simulink model "Deployed_On_CPU2"  (R2020a)
settings: Solver=ode4  StartTime=0.0  StopTime=Inf  FixedStep=0.01  RelTol=1e-3  EnableMultiTasking=on
undefined symbols (not defined in the file): C28x, CPU1, CPU2
libraries: c280xlib x47, dspobslib x27, simulink x20, c2837xDlib x1
(part 1 of 3)
settings Model: ExtModeTrigDuration=8  Creator=NRPU  LastModifiedBy=NRPU
settings DataIOCC: SaveFormat=Array
settings OptimizationCC: DefaultUnderspecifiedDataType=single  EnhancedBackFolding=on  PassReuseOutputArgsAs=Individual arguments  MaxStackSize=1024  OptimizeBlockOrder=speed  DifferentSizesBufferReuse=on  OptimizationCustomize=off  DenormalBehavior=FlushToZero  EfficientTunableParamExpr=on
settings DebuggingCC: ParameterTunabilityLossMsg=error
settings HardwareCC: ProdBitPerChar=16  ProdBitPerInt=16  ProdBitPerPointer=32  ProdBitPerSizeT=32  ProdBitPerPtrDiffT=32  ProdLargestAtomicInteger=Integer  ProdLargestAtomicFloat=None  ProdWordSize=16  ProdLongLongMode=on  ProdHWDeviceType=Texas Instruments->C2000
settings SFSimCC: SimCustomHeaderCode="#include \"MadgwickAHRS.h\""  SimCustomInitializer=intialize();  SimUserSources=MadgwickAHRS.c  SimAnalyzeCustomCode=on  MATLABDynamicMemAlloc=off
settings RTWCC: SystemTargetFile=ert.tlc  HardwareBoard=TI Delfino F28379D LaunchPad  TLCOptions=-aInlineSetEventsForThisBaseRateFcn=TLC_FALSE -aSuppressMultiTaskScheduler=TLC_FALSE -aRateBasedStepFcn=1  TemplateMakefile=ert_default_tmf  RTWUseSimCustomCode=on  CustomHeaderCode="#include \"MadgwickAHRS.h\""  CustomSource=MadgwickAHRS.c  CustomInitializer=intialize();  Toolchain=Texas Instruments Code Composer Studio (C2000)  BuildConfiguration=Specify
settings CodeAppCC: ForceParamTrailComments=on  IgnoreCustomStorageClasses=off  OperatorAnnotations=on  SimulinkDataObjDesc=on  SFDataObjDesc=on  InsertBlockDesc=on
settings ERTTargetCC: CodeReplacementLibrary=TI C28x  SupportContinuousTime=on  ExtModeStaticAllocSize=10000

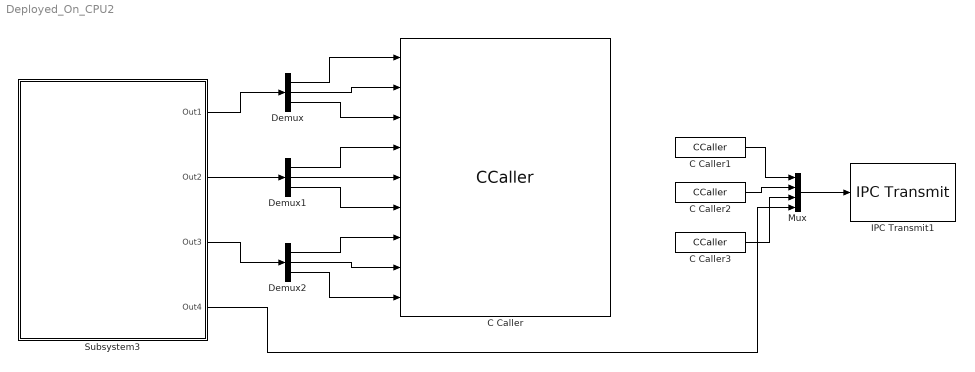
== system Deployed_On_CPU2 ==
  C Caller : CCaller  FunctionName=MadgwickQuaternionUpdate  PortSpecificationStruct="%)30     .    N!    8    (     @         %    \"     H    !     0         %  0 \"0    $    _    07)G3F%M90  4&]R=$YA;64 4V-O<&4     26YD97@     5'EP90      4VEZ90      27-';&]B86P   X    P    !@    @    $          4    (     0    ,    !         !   P!O=70 #@   #     &    \"     0         !0    @    !     P    $         $  # &]U=  .    .     8    (    !          %    \"     $    &     0         0   ...(+5398 chars)"
  C Caller1 : CCaller  FunctionName=roll  PortSpecificationStruct="%)30     .    & (   8    (     @         %    \"     $    !     0         %  0 \"0    $    _    07)G3F%M90  4&]R=$YA;64 4V-O<&4     26YD97@     5'EP90      4VEZ90      27-';&]B86P   X    P    !@    @    $          4    (     0    ,    !         !   P!O=70 #@   #     &    \"     0         !0    @    !     P    $         $  # &]U=  .    .     8    (    !          %    \"     $    &     0         0    !@   $]U='!U=   #@   #@    &    \"     8         !0    @    !     0    $         \"0    @               X    X    !@    @    $          4    (     0    8    !         !     &    <VEN9VQE   .    ,     8    (    !          %    \"     $    !     0         0  $ ,0    X    P    !@    @    ) @        4    (     0    $    !          (  0"
  C Caller2 : CCaller  FunctionName=pitch  PortSpecificationStruct="%)30     .    & (   8    (     @         %    \"     $    !     0         %  0 \"0    $    _    07)G3F%M90  4&]R=$YA;64 4V-O<&4     26YD97@     5'EP90      4VEZ90      27-';&]B86P   X    P    !@    @    $          4    (     0    ,    !         !   P!O=70 #@   #     &    \"     0         !0    @    !     P    $         $  # &]U=  .    .     8    (    !          %    \"     $    &     0         0    !@   $]U='!U=   #@   #@    &    \"     8         !0    @    !     0    $         \"0    @               X    X    !@    @    $          4    (     0    8    !         !     &    <VEN9VQE   .    ,     8    (    !          %    \"     $    !     0         0  $ ,0    X    P    !@    @    ) @        4    (     0    $    !          (  0"
  C Caller3 : CCaller  FunctionName=yaw  PortSpecificationStruct="%)30     .    & (   8    (     @         %    \"     $    !     0         %  0 \"0    $    _    07)G3F%M90  4&]R=$YA;64 4V-O<&4     26YD97@     5'EP90      4VEZ90      27-';&]B86P   X    P    !@    @    $          4    (     0    ,    !         !   P!O=70 #@   #     &    \"     0         !0    @    !     P    $         $  # &]U=  .    .     8    (    !          %    \"     $    &     0         0    !@   $]U='!U=   #@   #@    &    \"     8         !0    @    !     0    $         \"0    @               X    X    !@    @    $          4    (     0    8    !         !     &    <VEN9VQE   .    ,     8    (    !          %    \"     $    !     0         0  $ ,0    X    P    !@    @    ) @        4    (     0    $    !          (  0"
  Demux : Demux  Outputs=3
  Demux1 : Demux  Outputs=3
  Demux2 : Demux  Outputs=3
  IPC Transmit1 : c2837xDlib/IPC Transmit  blkParamProc=F2837x  SelectDestination=C28x (CPU1/CPU2)  SelectChannel=0  EnableBlocking=on
      settings: SourceProductBaseCode=TIC2000
  Mux : Mux
  Subsystem3 : Subsystem
      mask Display:
      | disp('GY-80')
      | port_label('Output',1,'Accelerometer','texmode','on')
      | port_label('Output',2,'Gyroscope','texmode','on')
      | port_label('Output',3,'Magnetometer','texmode','on')
      | port_label('Output',4,'MS5803','texmode','on')
  wires:
  Demux/1 -> C Caller/1
  Demux/2 -> C Caller/2
  Demux/3 -> C Caller/3
  Demux1/1 -> C Caller/4
  Demux1/2 -> C Caller/5
  Demux1/3 -> C Caller/6
  Demux2/1 -> C Caller/7
  Demux2/2 -> C Caller/8
  Demux2/3 -> C Caller/9
  C Caller1/1 -> Mux/1
  C Caller2/1 -> Mux/2
  C Caller3/1 -> Mux/3
  Subsystem3/1(Out1) -> Demux/1
  Subsystem3/2(Out2) -> Demux1/1
  Subsystem3/3(Out3) -> Demux2/1
  Subsystem3/4(Out4) -> Mux/4
  Mux/1 -> IPC Transmit1/1

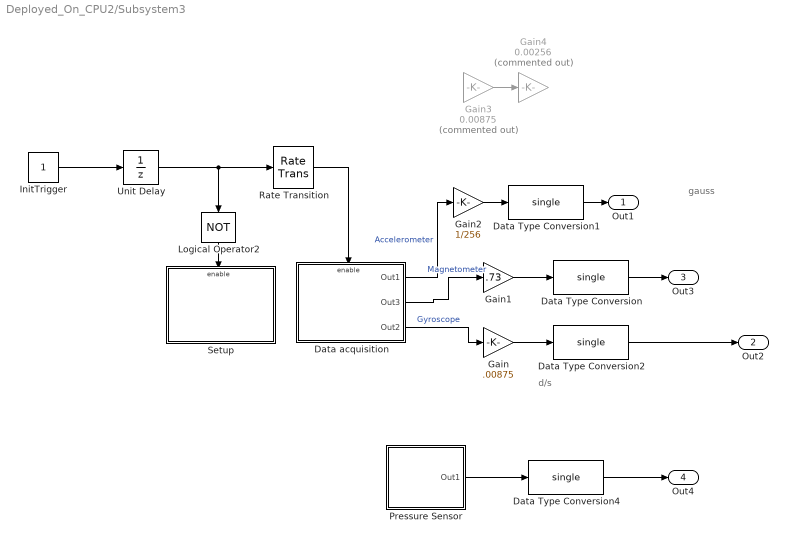
== system Deployed_On_CPU2/Subsystem3 ==
  note: gauss
  note: d/s
  Data Type Conversion{,1..2,4} (4 alike) : DataTypeConversion  OutDataTypeStr=single
  Data acquisition : Subsystem
  Gain : Gain  Gain=.00875  OutDataTypeStr=double
  Gain1 : Gain  Gain=.73  OutDataTypeStr=double
  Gain2 : Gain  Gain=1/256  OutDataTypeStr=double
  Gain3 : Gain  Commented=on  Gain=0.00875  OutDataTypeStr=int16
  Gain4 : Gain  Commented=on  Gain=0.00256  OutDataTypeStr=int16
  InitTrigger : Constant  Priority=10  OutDataTypeStr=uint16  SampleTime=0.01
  Logical Operator2 : Logic  Operator=NOT  AllPortsSameDT=off  OutDataTypeStr=boolean
  Pressure Sensor : Subsystem
  Rate Transition : RateTransition  OutPortSampleTime=0.01
  Setup : Subsystem  TreatAsAtomicUnit=on
  Unit Delay : UnitDelay  SampleTime=-1  HasFrameUpgradeWarning=on
  Out1 : Outport
  Out2 : Outport  Port=2
  Out3 : Outport  Port=3
  Out4 : Outport  Port=4
  wires:
  Rate Transition/1 -> Data acquisition/Enable
  Logical Operator2/1 -> Setup/Enable
  Unit Delay/1 -> Logical Operator2/1, Rate Transition/1
  InitTrigger/1 -> Unit Delay/1
  Data acquisition/1(Out1) -> Gain2/1  "Accelerometer"
  Data acquisition/3(Out2) -> Gain/1  "Gyroscope"
  Data acquisition/2(Out3) -> Gain1/1  "Magnetometer"
  Data Type Conversion/1 -> Out3/1
  Data Type Conversion1/1 -> Out1/1
  Gain1/1 -> Data Type Conversion/1
  Gain3/1 -> Gain4/1
  Gain2/1 -> Data Type Conversion1/1
  Gain/1 -> Data Type Conversion2/1
  Data Type Conversion2/1 -> Out2/1
  Pressure Sensor/1(Out1) -> Data Type Conversion4/1
  Data Type Conversion4/1 -> Out4/1

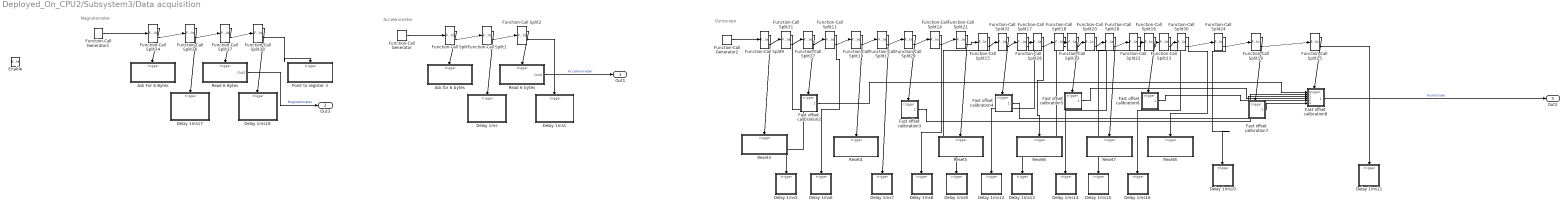
== system Deployed_On_CPU2/Subsystem3/Data acquisition ==
  note: Gyroscope
  note: Magnetometer
  note: Accelerometer
  Enable : EnablePort
  Ask For 6 Bytes : Subsystem  TreatAsAtomicUnit=on
  Ask for 6 bytes : Subsystem  TreatAsAtomicUnit=on
  Delay 1ms : Subsystem  TreatAsAtomicUnit=on
  Delay 1ms1 : Subsystem  TreatAsAtomicUnit=on
  Delay 1ms10 : Subsystem  TreatAsAtomicUnit=on
  Delay 1ms11 : Subsystem  TreatAsAtomicUnit=on
  Delay 1ms12 : Subsystem  TreatAsAtomicUnit=on
  Delay 1ms13 : Subsystem  TreatAsAtomicUnit=on
  Delay 1ms14 : Subsystem  TreatAsAtomicUnit=on
  Delay 1ms15 : Subsystem  TreatAsAtomicUnit=on
  Delay 1ms16 : Subsystem  TreatAsAtomicUnit=on
  Delay 1ms17 : Subsystem  TreatAsAtomicUnit=on
  Delay 1ms18 : Subsystem  TreatAsAtomicUnit=on
  Delay 1ms5 : Subsystem  TreatAsAtomicUnit=on
  Delay 1ms6 : Subsystem  TreatAsAtomicUnit=on
  Delay 1ms7 : Subsystem  TreatAsAtomicUnit=on
  Delay 1ms8 : Subsystem  TreatAsAtomicUnit=on
  Delay 1ms9 : Subsystem  TreatAsAtomicUnit=on
  Fast offset calibration2 : Subsystem  TreatAsAtomicUnit=on
  Fast offset calibration3 : Subsystem  TreatAsAtomicUnit=on
  Fast offset calibration4 : Subsystem  TreatAsAtomicUnit=on
  Fast offset calibration5 : Subsystem  TreatAsAtomicUnit=on
  Fast offset calibration6 : Subsystem  TreatAsAtomicUnit=on
  Fast offset calibration7 : Subsystem  TreatAsAtomicUnit=on
  Fast offset calibration8 : Subsystem  TreatAsAtomicUnit=on
  Function-Call Generator : simulink/Ports & Subsystems/Function-Call Generator  sample_time=0.01  numberOfIterations=1
  Function-Call Generator1 : simulink/Ports & Subsystems/Function-Call Generator  sample_time=0.01  numberOfIterations=1
  Function-Call Generator2 : simulink/Ports & Subsystems/Function-Call Generator  sample_time=0.01  numberOfIterations=1
  Function-Call Split{,1..2,9..32,34,36..38} (31 alike) : FunctionCallSplit  NumOutputPorts=2
  Ponit to register 3 : Subsystem  TreatAsAtomicUnit=on
  Read 6 Bytes : Subsystem  TreatAsAtomicUnit=on
  Read 6 bytes : Subsystem  TreatAsAtomicUnit=on
  Reset3 : Subsystem  TreatAsAtomicUnit=on
  Reset4 : Subsystem  TreatAsAtomicUnit=on
  Reset5 : Subsystem  TreatAsAtomicUnit=on
  Reset6 : Subsystem  TreatAsAtomicUnit=on
  Reset7 : Subsystem  TreatAsAtomicUnit=on
  Reset8 : Subsystem  TreatAsAtomicUnit=on
  Out1 : Outport
  Out3 : Outport  Port=2
  Out2 : Outport  Port=3
  wires:
  Function-Call Split19/2 -> Function-Call Split25/1
  Function-Call Split9/2 -> Function-Call Split31/1
  Function-Call Split27/1 -> Fast offset calibration2/Trigger
  Function-Call Split16/1 -> Fast offset calibration6/Trigger
  Function-Call Split10/2 -> Function-Call Split12/1
  Function-Call Split25/2 -> Delay 1ms11/Trigger
  Function-Call Split17/1 -> Delay 1ms12/Trigger
  Fast offset calibration7/1(Input) -> Fast offset calibration8/6(Input5)
  Fast offset calibration6/1(Input) -> Fast offset calibration8/5(Input4)
  Function-Call Split9/1 -> Reset3/Trigger
  Fast offset calibration2/1(Input) -> Fast offset calibration8/1(Input)
  Function-Call Split23/2 -> Function-Call Split30/1
  Fast offset calibration3/1(Input) -> Fast offset calibration8/2(Input1)
  Fast offset calibration4/1(Input) -> Fast offset calibration8/3(Input2)
  Function-Call Split32/2 -> Function-Call Split17/1
  Fast offset calibration8/1(Out2) -> Out2/1  "Gyroscope"
  Function-Call Split18/2 -> Function-Call Split13/1
  Function-Call Split24/1 -> Delay 1ms10/Trigger
  Function-Call Split10/1 -> Reset4/Trigger
  Function-Call Split29/2 -> Function-Call Split14/1
  Function-Call Split23/1 -> Delay 1ms16/Trigger
  Function-Call Split31/2 -> Function-Call Split27/1
  Function-Call Split17/2 -> Function-Call Split26/1
  Function-Call Split14/1 -> Delay 1ms8/Trigger
  Function-Call Split30/2 -> Function-Call Split24/1
  Function-Call Split21/1 -> Reset5/Trigger
  Function-Call Split30/1 -> Reset8/Trigger
  Function-Call Split11/2 -> Function-Call Split10/1
  Function-Call Split31/1 -> Delay 1ms5/Trigger
  Function-Call Split32/1 -> Fast offset calibration4/Trigger
  Fast offset calibration5/1(Input) -> Fast offset calibration8/4(Input3)
  Function-Call Split13/1 -> Fast offset calibration5/Trigger
  Function-Call Split15/2 -> Function-Call Split32/1
  Function-Call Split15/1 -> Delay 1ms9/Trigger
  Function-Call Split12/2 -> Function-Call Split29/1
  Function-Call Split20/2 -> Function-Call Split28/1
  Function-Call Split12/1 -> Delay 1ms7/Trigger
  Function-Call Split11/1 -> Delay 1ms6/Trigger
  Function-Call Split22/2 -> Function-Call Split16/1
  Function-Call Split26/1 -> Reset6/Trigger
  Function-Call Split28/2 -> Function-Call Split22/1
  Function-Call Split29/1 -> Fast offset calibration3/Trigger
  Function-Call Split20/1 -> Delay 1ms14/Trigger
  Function-Call Split22/1 -> Delay 1ms15/Trigger
  Function-Call Split13/2 -> Function-Call Split20/1
  Function-Call Split18/1 -> Delay 1ms13/Trigger
  Function-Call Split14/2 -> Function-Call Split21/1
  Function-Call Split21/2 -> Function-Call Split15/1
  Function-Call Split26/2 -> Function-Call Split18/1
  Function-Call Split19/1 -> Fast offset calibration7/Trigger
  Function-Call Split25/1 -> Fast offset calibration8/Trigger
  Function-Call Split27/2 -> Function-Call Split11/1
  Function-Call Split24/2 -> Function-Call Split19/1
  Function-Call Split28/1 -> Reset7/Trigger
  Function-Call Split16/2 -> Function-Call Split23/1
  Function-Call Split2/2 -> Delay 1ms1/Trigger
  Function-Call Split2/1 -> Read 6 bytes/Trigger
  Function-Call Split1/2 -> Function-Call Split2/1
  Function-Call Split/2 -> Function-Call Split1/1
  Function-Call Split1/1 -> Delay 1ms/Trigger
  Read 6 bytes/1(Out2) -> Out1/1  "Accelerometer"
  Function-Call Generator/1 -> Function-Call Split/1
  Function-Call Split/1 -> Ask for 6 bytes/Trigger
  Function-Call Split36/2 -> Function-Call Split37/1
  Function-Call Split37/2 -> Function-Call Split38/1
  Function-Call Split38/1 -> Delay 1ms18/Trigger
  Function-Call Generator1/1 -> Function-Call Split34/1
  Function-Call Split36/1 -> Delay 1ms17/Trigger
  Read 6 Bytes/1(Out2) -> Out3/1  "Magnetometer"
  Function-Call Split34/2 -> Function-Call Split36/1
  Function-Call Split37/1 -> Read 6 Bytes/Trigger
  Function-Call Split34/1 -> Ask For 6 Bytes/Trigger
  Function-Call Split38/2 -> Ponit to register 3/Trigger
  Function-Call Generator2/1 -> Function-Call Split9/1

== system Deployed_On_CPU2/Subsystem3/Pressure Sensor ==
  Data acquisition : Subsystem  Commented=on
  InitTrigger : Constant  Priority=10  Commented=on  OutDataTypeStr=uint16  SampleTime=0.01
  Logical Operator2 : Logic  Commented=on  Operator=NOT  AllPortsSameDT=off  OutDataTypeStr=boolean
  Rate Transition : RateTransition  Commented=on  OutPortSampleTime=0.01
  Setup : Subsystem  Commented=on  TreatAsAtomicUnit=on
  Unit Delay : UnitDelay  Commented=on  SampleTime=-1  HasFrameUpgradeWarning=on
  Out1 : Outport
  wires:
  Unit Delay/1 -> Logical Operator2/1, Rate Transition/1
  Data acquisition/1(Out1) -> Out1/1
  Rate Transition/1 -> Data acquisition/Enable
  InitTrigger/1 -> Unit Delay/1
  Logical Operator2/1 -> Setup/Enable

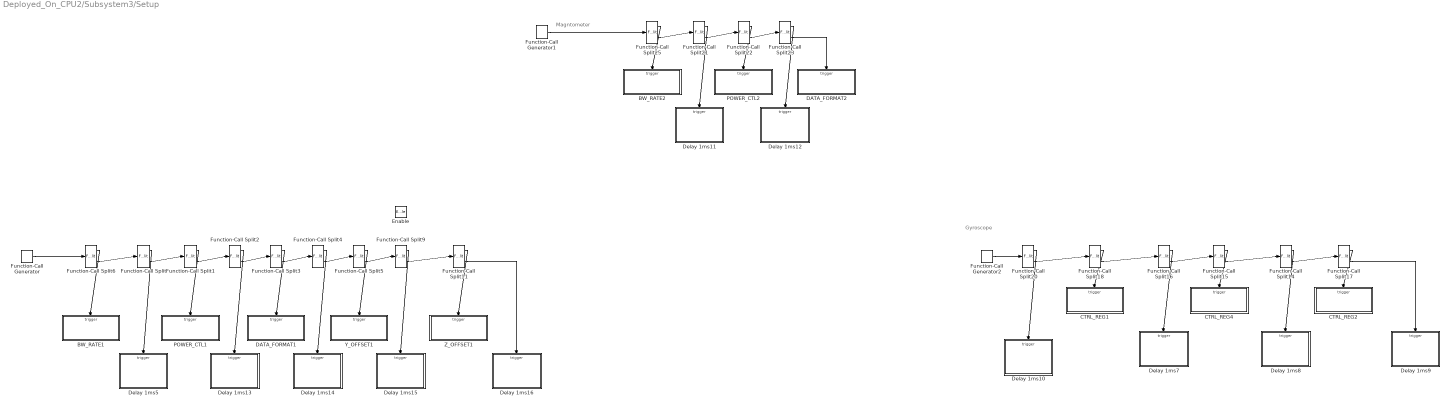
== system Deployed_On_CPU2/Subsystem3/Setup ==
  note: Gyroscope
  note: Magntometer
  Enable : EnablePort
  BW_RATE1 : Subsystem  TreatAsAtomicUnit=on
  BW_RATE2 : Subsystem  TreatAsAtomicUnit=on
  CTRL_REG1 : Subsystem  TreatAsAtomicUnit=on
  CTRL_REG2 : Subsystem  TreatAsAtomicUnit=on
  CTRL_REG4 : Subsystem  TreatAsAtomicUnit=on
  DATA_FORMAT1 : Subsystem  TreatAsAtomicUnit=on
  DATA_FORMAT2 : Subsystem  TreatAsAtomicUnit=on
  Delay 1ms10 : Subsystem  TreatAsAtomicUnit=on
  Delay 1ms11 : Subsystem  TreatAsAtomicUnit=on
  Delay 1ms12 : Subsystem  TreatAsAtomicUnit=on
  Delay 1ms13 : Subsystem  TreatAsAtomicUnit=on
  Delay 1ms14 : Subsystem  TreatAsAtomicUnit=on
  Delay 1ms15 : Subsystem  TreatAsAtomicUnit=on
  Delay 1ms16 : Subsystem  TreatAsAtomicUnit=on
  Delay 1ms5 : Subsystem  TreatAsAtomicUnit=on
  Delay 1ms7 : Subsystem  TreatAsAtomicUnit=on
  Delay 1ms8 : Subsystem  TreatAsAtomicUnit=on
  Delay 1ms9 : Subsystem  TreatAsAtomicUnit=on
  Function-Call Generator : simulink/Ports & Subsystems/Function-Call Generator  sample_time=0.01  numberOfIterations=1
  Function-Call Generator1 : simulink/Ports & Subsystems/Function-Call Generator  sample_time=0.01  numberOfIterations=1
  Function-Call Generator2 : simulink/Ports & Subsystems/Function-Call Generator  sample_time=0.01  numberOfIterations=1
  Function-Call Split{,1..6,9,11,14..18,20..23,25} (19 alike) : FunctionCallSplit  NumOutputPorts=2
  POWER_CTL1 : Subsystem  TreatAsAtomicUnit=on
  POWER_CTL2 : Subsystem  TreatAsAtomicUnit=on
  Y_OFFSET1 : Subsystem  TreatAsAtomicUnit=on
  Z_OFFSET1 : Subsystem  TreatAsAtomicUnit=on
  wires:
  Function-Call Split20/1 -> Delay 1ms10/Trigger
  Function-Call Split17/2 -> Delay 1ms9/Trigger
  Function-Call Split15/1 -> CTRL_REG4/Trigger
  Function-Call Split15/2 -> Function-Call Split14/1
  Function-Call Split16/2 -> Function-Call Split15/1
  Function-Call Split17/1 -> CTRL_REG2/Trigger
  Function-Call Split14/2 -> Function-Call Split17/1
  Function-Call Split18/1 -> CTRL_REG1/Trigger
  Function-Call Split20/2 -> Function-Call Split18/1
  Function-Call Split14/1 -> Delay 1ms8/Trigger
  Function-Call Split16/1 -> Delay 1ms7/Trigger
  Function-Call Split18/2 -> Function-Call Split16/1
  Function-Call Split3/2 -> Function-Call Split4/1
  Function-Call Split4/2 -> Function-Call Split5/1
  Function-Call Split2/2 -> Function-Call Split3/1
  Function-Call Split/2 -> Function-Call Split1/1
  Function-Call Split1/2 -> Function-Call Split2/1
  Function-Call Split23/2 -> DATA_FORMAT2/Trigger
  Function-Call Split21/2 -> Function-Call Split22/1
  Function-Call Split21/1 -> Delay 1ms11/Trigger
  Function-Call Split23/1 -> Delay 1ms12/Trigger
  Function-Call Split22/2 -> Function-Call Split23/1
  Function-Call Split25/2 -> Function-Call Split21/1
  Function-Call Split25/1 -> BW_RATE2/Trigger
  Function-Call Split22/1 -> POWER_CTL2/Trigger
  Function-Call Generator1/1 -> Function-Call Split25/1
  Function-Call Generator2/1 -> Function-Call Split20/1
  Function-Call Split5/2 -> Function-Call Split9/1
  Function-Call Split9/2 -> Function-Call Split11/1
  Function-Call Split/1 -> Delay 1ms5/Trigger
  Function-Call Split4/1 -> Delay 1ms14/Trigger
  Function-Call Split9/1 -> Delay 1ms15/Trigger
  Function-Call Split2/1 -> Delay 1ms13/Trigger
  Function-Call Split11/2 -> Delay 1ms16/Trigger
  Function-Call Split1/1 -> POWER_CTL1/Trigger
  Function-Call Split3/1 -> DATA_FORMAT1/Trigger
  Function-Call Split5/1 -> Y_OFFSET1/Trigger
  Function-Call Split11/1 -> Z_OFFSET1/Trigger
  Function-Call Split6/1 -> BW_RATE1/Trigger
  Function-Call Split6/2 -> Function-Call Split/1
  Function-Call Generator/1 -> Function-Call Split6/1

== system Deployed_On_CPU2/Subsystem3/Data acquisition/Ask For 6 Bytes ==
  function : TriggerPort  TriggerType=function-call  VariantControl=Variant
  Data Read Adress : Constant  Priority=10  Value=hex2dec('06')  OutDataTypeStr=uint8  SampleTime=-1
  I2C Transmit : c280xlib/I2C Transmit  Priority=20  selectModule=I2C_A  addrFormat=7-Bit addressing  saSource=Specify via dialog  SAR=hex2dec('1E')  bitCount=8  STP=on  RM=off  STR=on
      settings: SourceProductBaseCode=TIC2000
  Terminator : Terminator
  wires:
  Data Read Adress/1 -> I2C Transmit/1
  I2C Transmit/1 -> Terminator/1

== system Deployed_On_CPU2/Subsystem3/Data acquisition/Ask for 6 bytes ==
  function : TriggerPort  TriggerType=function-call  VariantControl=Variant
  Data Read Adress : Constant  Priority=10  Value=hex2dec('32')  OutDataTypeStr=uint8  SampleTime=-1
  I2C Transmit : c280xlib/I2C Transmit  Priority=20  selectModule=I2C_A  addrFormat=7-Bit addressing  saSource=Specify via dialog  SAR=83  bitCount=8  STP=on  RM=off  STR=on
      settings: SourceProductBaseCode=TIC2000
  Terminator : Terminator
  wires:
  I2C Transmit/1 -> Terminator/1
  Data Read Adress/1 -> I2C Transmit/1

== system Deployed_On_CPU2/Subsystem3/Data acquisition/Delay 1ms ==
  function : TriggerPort  TriggerType=function-call  VariantControl=Variant
  System Outputs : Subsystem  mask(System Outputs){ShowInLibBrowser=0}
      mask prompts: ShowInLibBrowser "Simulink:masks:CustCodeMaskParam1_MP"
      settings: CopyFcn=cccopyfcn(gcb)  OpenFcn=ccopenfcn('System Outputs Function')
      mask Help: eval('feval(''rtwprivate'',''rtwhelpview'',''rtw_sys_outputs_block'')');
      mask Display: disp('System\nOutputs');

== system Deployed_On_CPU2/Subsystem3/Data acquisition/Delay 1ms1 ==
  function : TriggerPort  TriggerType=function-call  VariantControl=Variant
  System Outputs : Subsystem  mask(System Outputs){ShowInLibBrowser=0}
      mask prompts: ShowInLibBrowser "Simulink:masks:CustCodeMaskParam1_MP"
      settings: CopyFcn=cccopyfcn(gcb)  OpenFcn=ccopenfcn('System Outputs Function')
      mask Help: eval('feval(''rtwprivate'',''rtwhelpview'',''rtw_sys_outputs_block'')');
      mask Display: disp('System\nOutputs');

== system Deployed_On_CPU2/Subsystem3/Data acquisition/Delay 1ms10 ==
  function : TriggerPort  TriggerType=function-call  VariantControl=Variant
  System Outputs : Subsystem  mask(System Outputs){ShowInLibBrowser=0}
      mask prompts: ShowInLibBrowser "Simulink:masks:CustCodeMaskParam1_MP"
      settings: CopyFcn=cccopyfcn(gcb)  OpenFcn=ccopenfcn('System Outputs Function')
      mask Help: eval('feval(''rtwprivate'',''rtwhelpview'',''rtw_sys_outputs_block'')');
      mask Display: disp('System\nOutputs');

== system Deployed_On_CPU2/Subsystem3/Data acquisition/Delay 1ms11 ==
  function : TriggerPort  TriggerType=function-call  VariantControl=Variant
  System Outputs : Subsystem  mask(System Outputs){ShowInLibBrowser=0}
      mask prompts: ShowInLibBrowser "Simulink:masks:CustCodeMaskParam1_MP"
      settings: CopyFcn=cccopyfcn(gcb)  OpenFcn=ccopenfcn('System Outputs Function')
      mask Help: eval('feval(''rtwprivate'',''rtwhelpview'',''rtw_sys_outputs_block'')');
      mask Display: disp('System\nOutputs');

== system Deployed_On_CPU2/Subsystem3/Data acquisition/Delay 1ms12 ==
  function : TriggerPort  TriggerType=function-call  VariantControl=Variant
  System Outputs : Subsystem  mask(System Outputs){ShowInLibBrowser=0}
      mask prompts: ShowInLibBrowser "Simulink:masks:CustCodeMaskParam1_MP"
      settings: CopyFcn=cccopyfcn(gcb)  OpenFcn=ccopenfcn('System Outputs Function')
      mask Help: eval('feval(''rtwprivate'',''rtwhelpview'',''rtw_sys_outputs_block'')');
      mask Display: disp('System\nOutputs');

== system Deployed_On_CPU2/Subsystem3/Data acquisition/Delay 1ms13 ==
  function : TriggerPort  TriggerType=function-call  VariantControl=Variant
  System Outputs : Subsystem  mask(System Outputs){ShowInLibBrowser=0}
      mask prompts: ShowInLibBrowser "Simulink:masks:CustCodeMaskParam1_MP"
      settings: CopyFcn=cccopyfcn(gcb)  OpenFcn=ccopenfcn('System Outputs Function')
      mask Help: eval('feval(''rtwprivate'',''rtwhelpview'',''rtw_sys_outputs_block'')');
      mask Display: disp('System\nOutputs');

== system Deployed_On_CPU2/Subsystem3/Data acquisition/Delay 1ms14 ==
  function : TriggerPort  TriggerType=function-call  VariantControl=Variant
  System Outputs : Subsystem  mask(System Outputs){ShowInLibBrowser=0}
      mask prompts: ShowInLibBrowser "Simulink:masks:CustCodeMaskParam1_MP"
      settings: CopyFcn=cccopyfcn(gcb)  OpenFcn=ccopenfcn('System Outputs Function')
      mask Help: eval('feval(''rtwprivate'',''rtwhelpview'',''rtw_sys_outputs_block'')');
      mask Display: disp('System\nOutputs');

== system Deployed_On_CPU2/Subsystem3/Data acquisition/Delay 1ms15 ==
  function : TriggerPort  TriggerType=function-call  VariantControl=Variant
  System Outputs : Subsystem  mask(System Outputs){ShowInLibBrowser=0}
      mask prompts: ShowInLibBrowser "Simulink:masks:CustCodeMaskParam1_MP"
      settings: CopyFcn=cccopyfcn(gcb)  OpenFcn=ccopenfcn('System Outputs Function')
      mask Help: eval('feval(''rtwprivate'',''rtwhelpview'',''rtw_sys_outputs_block'')');
      mask Display: disp('System\nOutputs');

== system Deployed_On_CPU2/Subsystem3/Data acquisition/Delay 1ms16 ==
  function : TriggerPort  TriggerType=function-call  VariantControl=Variant
  System Outputs : Subsystem  mask(System Outputs){ShowInLibBrowser=0}
      mask prompts: ShowInLibBrowser "Simulink:masks:CustCodeMaskParam1_MP"
      settings: CopyFcn=cccopyfcn(gcb)  OpenFcn=ccopenfcn('System Outputs Function')
      mask Help: eval('feval(''rtwprivate'',''rtwhelpview'',''rtw_sys_outputs_block'')');
      mask Display: disp('System\nOutputs');

== system Deployed_On_CPU2/Subsystem3/Data acquisition/Delay 1ms17 ==
  function : TriggerPort  TriggerType=function-call  VariantControl=Variant
  System Outputs : Subsystem  mask(System Outputs){ShowInLibBrowser=0}
      mask prompts: ShowInLibBrowser "Simulink:masks:CustCodeMaskParam1_MP"
      settings: CopyFcn=cccopyfcn(gcb)  OpenFcn=ccopenfcn('System Outputs Function')
      mask Help: eval('feval(''rtwprivate'',''rtwhelpview'',''rtw_sys_outputs_block'')');
      mask Display: disp('System\nOutputs');

== system Deployed_On_CPU2/Subsystem3/Data acquisition/Delay 1ms18 ==
  function : TriggerPort  TriggerType=function-call  VariantControl=Variant
  System Outputs : Subsystem  mask(System Outputs){ShowInLibBrowser=0}
      mask prompts: ShowInLibBrowser "Simulink:masks:CustCodeMaskParam1_MP"
      settings: CopyFcn=cccopyfcn(gcb)  OpenFcn=ccopenfcn('System Outputs Function')
      mask Help: eval('feval(''rtwprivate'',''rtwhelpview'',''rtw_sys_outputs_block'')');
      mask Display: disp('System\nOutputs');

== system Deployed_On_CPU2/Subsystem3/Data acquisition/Delay 1ms5 ==
  function : TriggerPort  TriggerType=function-call  VariantControl=Variant
  System Outputs : Subsystem  mask(System Outputs){ShowInLibBrowser=0}
      mask prompts: ShowInLibBrowser "Simulink:masks:CustCodeMaskParam1_MP"
      settings: CopyFcn=cccopyfcn(gcb)  OpenFcn=ccopenfcn('System Outputs Function')
      mask Help: eval('feval(''rtwprivate'',''rtwhelpview'',''rtw_sys_outputs_block'')');
      mask Display: disp('System\nOutputs');

== system Deployed_On_CPU2/Subsystem3/Data acquisition/Delay 1ms6 ==
  function : TriggerPort  TriggerType=function-call  VariantControl=Variant
  System Outputs : Subsystem  mask(System Outputs){ShowInLibBrowser=0}
      mask prompts: ShowInLibBrowser "Simulink:masks:CustCodeMaskParam1_MP"
      settings: CopyFcn=cccopyfcn(gcb)  OpenFcn=ccopenfcn('System Outputs Function')
      mask Help: eval('feval(''rtwprivate'',''rtwhelpview'',''rtw_sys_outputs_block'')');
      mask Display: disp('System\nOutputs');

== system Deployed_On_CPU2/Subsystem3/Data acquisition/Delay 1ms7 ==
  function : TriggerPort  TriggerType=function-call  VariantControl=Variant
  System Outputs : Subsystem  mask(System Outputs){ShowInLibBrowser=0}
      mask prompts: ShowInLibBrowser "Simulink:masks:CustCodeMaskParam1_MP"
      settings: CopyFcn=cccopyfcn(gcb)  OpenFcn=ccopenfcn('System Outputs Function')
      mask Help: eval('feval(''rtwprivate'',''rtwhelpview'',''rtw_sys_outputs_block'')');
      mask Display: disp('System\nOutputs');

== system Deployed_On_CPU2/Subsystem3/Data acquisition/Delay 1ms8 ==
  function : TriggerPort  TriggerType=function-call  VariantControl=Variant
  System Outputs : Subsystem  mask(System Outputs){ShowInLibBrowser=0}
      mask prompts: ShowInLibBrowser "Simulink:masks:CustCodeMaskParam1_MP"
      settings: CopyFcn=cccopyfcn(gcb)  OpenFcn=ccopenfcn('System Outputs Function')
      mask Help: eval('feval(''rtwprivate'',''rtwhelpview'',''rtw_sys_outputs_block'')');
      mask Display: disp('System\nOutputs');

== system Deployed_On_CPU2/Subsystem3/Data acquisition/Delay 1ms9 ==
  function : TriggerPort  TriggerType=function-call  VariantControl=Variant
  System Outputs : Subsystem  mask(System Outputs){ShowInLibBrowser=0}
      mask prompts: ShowInLibBrowser "Simulink:masks:CustCodeMaskParam1_MP"
      settings: CopyFcn=cccopyfcn(gcb)  OpenFcn=ccopenfcn('System Outputs Function')
      mask Help: eval('feval(''rtwprivate'',''rtwhelpview'',''rtw_sys_outputs_block'')');
      mask Display: disp('System\nOutputs');

== system Deployed_On_CPU2/Subsystem3/Data acquisition/Fast offset calibration2 ==
  function : TriggerPort  TriggerType=function-call  VariantControl=Variant
  I2C Receive1 : c280xlib/I2C Receive  Priority=10  selectModule=I2C_A  addrFormat=7-Bit addressing  saSource=Specify via dialog  SAR=hex2dec('69')  bitCount=8  dataLength=1  initValue=0  NACK=off  STP=on  STR=on  sampleTime=-1  dataType=uint8
      settings: SourceProductBaseCode=TIC2000
  Terminator : Terminator
  Input : Outport
  wires:
  I2C Receive1/1 -> Input/1
  I2C Receive1/2 -> Terminator/1

== system Deployed_On_CPU2/Subsystem3/Data acquisition/Fast offset calibration3 ==
  function : TriggerPort  TriggerType=function-call  VariantControl=Variant
  I2C Receive1 : c280xlib/I2C Receive  Priority=10  selectModule=I2C_A  addrFormat=7-Bit addressing  saSource=Specify via dialog  SAR=hex2dec('69')  bitCount=8  dataLength=1  initValue=0  NACK=off  STP=on  STR=on  sampleTime=-1  dataType=uint8
      settings: SourceProductBaseCode=TIC2000
  Terminator : Terminator
  Input : Outport
  wires:
  I2C Receive1/2 -> Terminator/1
  I2C Receive1/1 -> Input/1

== system Deployed_On_CPU2/Subsystem3/Data acquisition/Fast offset calibration4 ==
  function : TriggerPort  TriggerType=function-call  VariantControl=Variant
  I2C Receive1 : c280xlib/I2C Receive  Priority=10  selectModule=I2C_A  addrFormat=7-Bit addressing  saSource=Specify via dialog  SAR=hex2dec('69')  bitCount=8  dataLength=1  initValue=0  NACK=off  STP=on  STR=on  sampleTime=-1  dataType=uint8
      settings: SourceProductBaseCode=TIC2000
  Terminator : Terminator
  Input : Outport
  wires:
  I2C Receive1/2 -> Terminator/1
  I2C Receive1/1 -> Input/1

== system Deployed_On_CPU2/Subsystem3/Data acquisition/Fast offset calibration5 ==
  function : TriggerPort  TriggerType=function-call  VariantControl=Variant
  I2C Receive1 : c280xlib/I2C Receive  Priority=10  selectModule=I2C_A  addrFormat=7-Bit addressing  saSource=Specify via dialog  SAR=hex2dec('69')  bitCount=8  dataLength=1  initValue=0  NACK=off  STP=on  STR=on  sampleTime=-1  dataType=uint8
      settings: SourceProductBaseCode=TIC2000
  Terminator : Terminator
  Input : Outport
  wires:
  I2C Receive1/2 -> Terminator/1
  I2C Receive1/1 -> Input/1

== system Deployed_On_CPU2/Subsystem3/Data acquisition/Fast offset calibration6 ==
  function : TriggerPort  TriggerType=function-call  VariantControl=Variant
  I2C Receive1 : c280xlib/I2C Receive  Priority=10  selectModule=I2C_A  addrFormat=7-Bit addressing  saSource=Specify via dialog  SAR=hex2dec('69')  bitCount=8  dataLength=1  initValue=0  NACK=off  STP=on  STR=on  sampleTime=-1  dataType=uint8
      settings: SourceProductBaseCode=TIC2000
  Terminator : Terminator
  Input : Outport
  wires:
  I2C Receive1/2 -> Terminator/1
  I2C Receive1/1 -> Input/1

== system Deployed_On_CPU2/Subsystem3/Data acquisition/Fast offset calibration7 ==
  function : TriggerPort  TriggerType=function-call  VariantControl=Variant
  I2C Receive1 : c280xlib/I2C Receive  Priority=10  selectModule=I2C_A  addrFormat=7-Bit addressing  saSource=Specify via dialog  SAR=hex2dec('69')  bitCount=8  dataLength=1  initValue=0  NACK=off  STP=on  STR=on  sampleTime=-1  dataType=uint8
      settings: SourceProductBaseCode=TIC2000
  Terminator : Terminator
  Input : Outport
  wires:
  I2C Receive1/2 -> Terminator/1
  I2C Receive1/1 -> Input/1

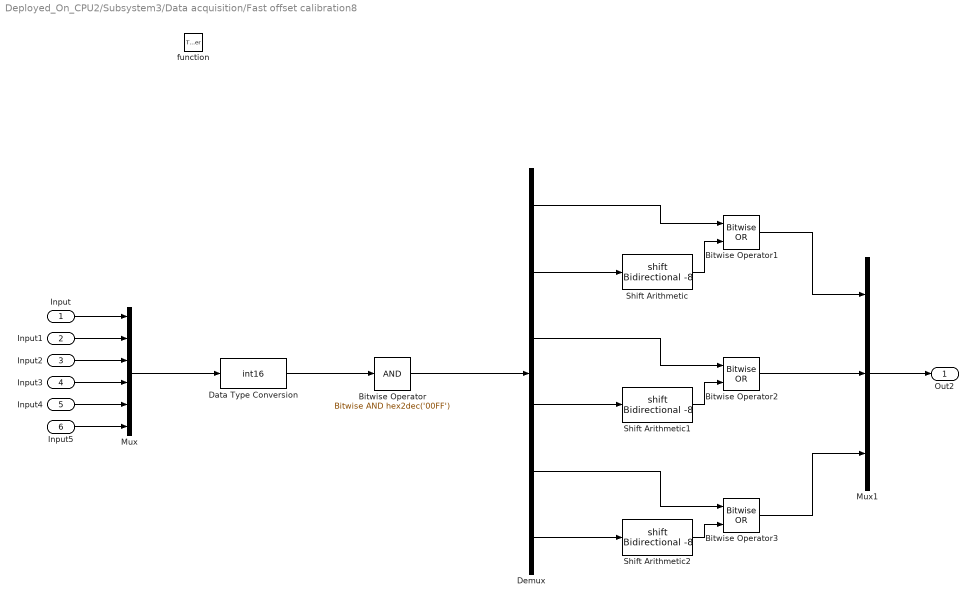
== system Deployed_On_CPU2/Subsystem3/Data acquisition/Fast offset calibration8 ==
  Input : Inport
  Input1 : Inport  Port=2
  Input2 : Inport  Port=3
  Input3 : Inport  Port=4
  Input4 : Inport  Port=5
  Input5 : Inport  Port=6
  function : TriggerPort  TriggerType=function-call  VariantControl=Variant
  Bitwise Operator : simulink/Logic and Bit Operations/Bitwise Operator  logicop=AND  UseBitMask=on  BitMask=hex2dec('00FF')  BitMaskRealWorld=Stored Integer
  Bitwise Operator1 : simulink/Logic and Bit Operations/Bitwise Operator  logicop=OR  UseBitMask=off  NumInputPorts=2  BitMask=bin2dec('11011001')  BitMaskRealWorld=Stored Integer
  Bitwise Operator2 : simulink/Logic and Bit Operations/Bitwise Operator  logicop=OR  UseBitMask=off  NumInputPorts=2  BitMask=bin2dec('11011001')  BitMaskRealWorld=Stored Integer
  Bitwise Operator3 : simulink/Logic and Bit Operations/Bitwise Operator  logicop=OR  UseBitMask=off  NumInputPorts=2  BitMask=bin2dec('11011001')  BitMaskRealWorld=Stored Integer
  Data Type Conversion : DataTypeConversion  OutDataTypeStr=int16  ConvertRealWorld=Stored Integer (SI)
  Demux : Demux  Outputs=6
  Mux : Mux  Inputs=6
  Mux1 : Mux  Inputs=3
  Shift Arithmetic : ArithShift  BitShiftNumber=-8
  Shift Arithmetic1 : ArithShift  BitShiftNumber=-8
  Shift Arithmetic2 : ArithShift  BitShiftNumber=-8
  Out2 : Outport
  wires:
  Demux/6 -> Shift Arithmetic2/1
  Input5/1 -> Mux/6
  Input4/1 -> Mux/5
  Input3/1 -> Mux/4
  Input2/1 -> Mux/3
  Input1/1 -> Mux/2
  Input/1 -> Mux/1
  Shift Arithmetic1/1 -> Bitwise Operator2/2
  Bitwise Operator2/1 -> Mux1/2
  Bitwise Operator3/1 -> Mux1/3
  Bitwise Operator1/1 -> Mux1/1
  Mux1/1 -> Out2/1
  Shift Arithmetic/1 -> Bitwise Operator1/2
  Demux/3 -> Bitwise Operator2/1
  Bitwise Operator/1 -> Demux/1
  Shift Arithmetic2/1 -> Bitwise Operator3/2
  Demux/5 -> Bitwise Operator3/1
  Demux/1 -> Bitwise Operator1/1
  Demux/2 -> Shift Arithmetic/1
  Data Type Conversion/1 -> Bitwise Operator/1
  Demux/4 -> Shift Arithmetic1/1
  Mux/1 -> Data Type Conversion/1

== system Deployed_On_CPU2/Subsystem3/Data acquisition/Ponit to register 3 ==
  function : TriggerPort  TriggerType=function-call  VariantControl=Variant
  Data Read Adress : Constant  Priority=10  Value=hex2dec('03')  OutDataTypeStr=uint8  SampleTime=-1
  I2C Transmit : c280xlib/I2C Transmit  Priority=20  selectModule=I2C_A  addrFormat=7-Bit addressing  saSource=Specify via dialog  SAR=hex2dec('1E')  bitCount=8  STP=on  RM=off  STR=on
      settings: SourceProductBaseCode=TIC2000
  Terminator : Terminator
  wires:
  I2C Transmit/1 -> Terminator/1
  Data Read Adress/1 -> I2C Transmit/1

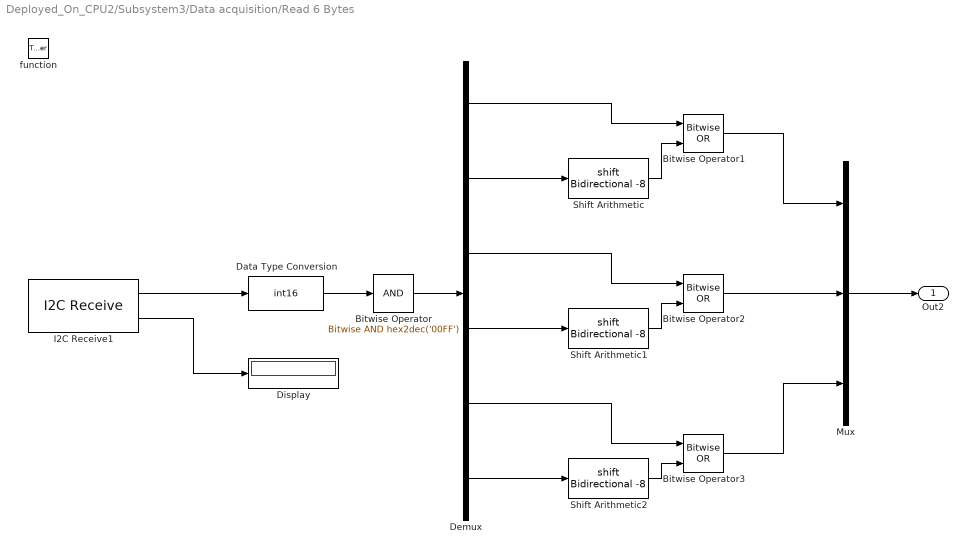
== system Deployed_On_CPU2/Subsystem3/Data acquisition/Read 6 Bytes ==
  function : TriggerPort  TriggerType=function-call  VariantControl=Variant
  Bitwise Operator : simulink/Logic and Bit Operations/Bitwise Operator  logicop=AND  UseBitMask=on  BitMask=hex2dec('00FF')  BitMaskRealWorld=Stored Integer
  Bitwise Operator1 : simulink/Logic and Bit Operations/Bitwise Operator  logicop=OR  UseBitMask=off  NumInputPorts=2  BitMask=bin2dec('11011001')  BitMaskRealWorld=Stored Integer
  Bitwise Operator2 : simulink/Logic and Bit Operations/Bitwise Operator  logicop=OR  UseBitMask=off  NumInputPorts=2  BitMask=bin2dec('11011001')  BitMaskRealWorld=Stored Integer
  Bitwise Operator3 : simulink/Logic and Bit Operations/Bitwise Operator  logicop=OR  UseBitMask=off  NumInputPorts=2  BitMask=bin2dec('11011001')  BitMaskRealWorld=Stored Integer
  Data Type Conversion : DataTypeConversion  OutDataTypeStr=int16  ConvertRealWorld=Stored Integer (SI)
  Demux : Demux  Outputs=6
  Display : Display
  I2C Receive1 : c280xlib/I2C Receive  Priority=10  selectModule=I2C_A  addrFormat=7-Bit addressing  saSource=Specify via dialog  SAR=hex2dec('1E')  bitCount=8  dataLength=6  initValue=0  NACK=off  STP=on  STR=on  sampleTime=-1  dataType=uint8
      settings: SourceProductBaseCode=TIC2000
  Mux : Mux  Inputs=3
  Shift Arithmetic : ArithShift  BitShiftNumber=-8
  Shift Arithmetic1 : ArithShift  BitShiftNumber=-8
  Shift Arithmetic2 : ArithShift  BitShiftNumber=-8
  Out2 : Outport
  wires:
  I2C Receive1/1 -> Data Type Conversion/1
  I2C Receive1/2 -> Display/1
  Data Type Conversion/1 -> Bitwise Operator/1
  Bitwise Operator/1 -> Demux/1
  Demux/5 -> Bitwise Operator3/1
  Demux/1 -> Bitwise Operator1/1
  Demux/6 -> Shift Arithmetic2/1
  Demux/4 -> Shift Arithmetic1/1
  Demux/2 -> Shift Arithmetic/1
  Shift Arithmetic2/1 -> Bitwise Operator3/2
  Shift Arithmetic1/1 -> Bitwise Operator2/2
  Demux/3 -> Bitwise Operator2/1
  Mux/1 -> Out2/1
  Shift Arithmetic/1 -> Bitwise Operator1/2
  Bitwise Operator2/1 -> Mux/2
  Bitwise Operator3/1 -> Mux/3
  Bitwise Operator1/1 -> Mux/1

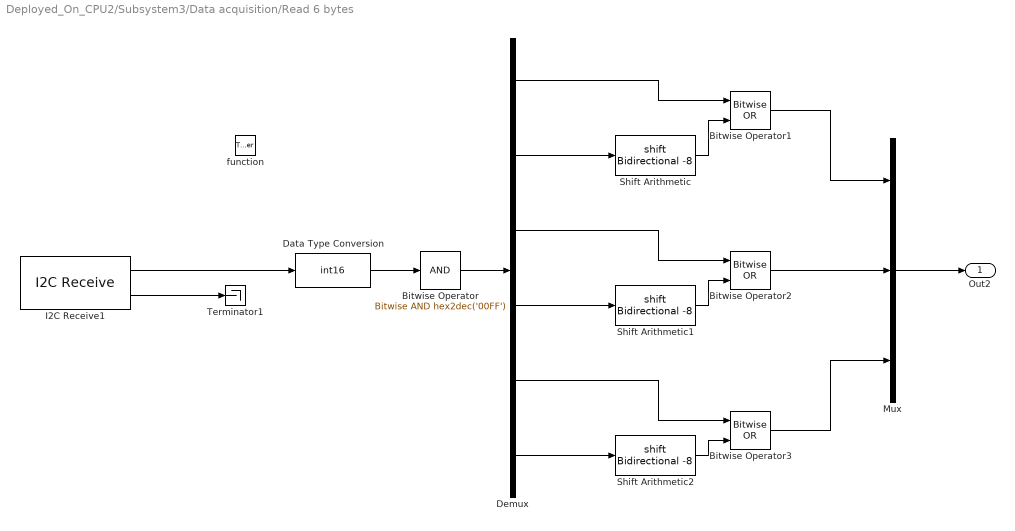
== system Deployed_On_CPU2/Subsystem3/Data acquisition/Read 6 bytes ==
  function : TriggerPort  TriggerType=function-call  VariantControl=Variant
  Bitwise Operator : simulink/Logic and Bit Operations/Bitwise Operator  logicop=AND  UseBitMask=on  BitMask=hex2dec('00FF')  BitMaskRealWorld=Stored Integer
  Bitwise Operator1 : simulink/Logic and Bit Operations/Bitwise Operator  logicop=OR  UseBitMask=off  NumInputPorts=2  BitMask=bin2dec('11011001')  BitMaskRealWorld=Stored Integer
  Bitwise Operator2 : simulink/Logic and Bit Operations/Bitwise Operator  logicop=OR  UseBitMask=off  NumInputPorts=2  BitMask=bin2dec('11011001')  BitMaskRealWorld=Stored Integer
  Bitwise Operator3 : simulink/Logic and Bit Operations/Bitwise Operator  logicop=OR  UseBitMask=off  NumInputPorts=2  BitMask=bin2dec('11011001')  BitMaskRealWorld=Stored Integer
  Data Type Conversion : DataTypeConversion  OutDataTypeStr=int16  ConvertRealWorld=Stored Integer (SI)
  Demux : Demux  Outputs=6
  I2C Receive1 : c280xlib/I2C Receive  Priority=10  selectModule=I2C_A  addrFormat=7-Bit addressing  saSource=Specify via dialog  SAR=83  bitCount=8  dataLength=6  initValue=0  NACK=off  STP=on  STR=on  sampleTime=-1  dataType=uint8
      settings: SourceProductBaseCode=TIC2000
  Mux : Mux  Inputs=3
  Shift Arithmetic : ArithShift  BitShiftNumber=-8
  Shift Arithmetic1 : ArithShift  BitShiftNumber=-8
  Shift Arithmetic2 : ArithShift  BitShiftNumber=-8
  Terminator1 : Terminator
  Out2 : Outport
  wires:
  Bitwise Operator1/1 -> Mux/1
  Bitwise Operator3/1 -> Mux/3
  Bitwise Operator2/1 -> Mux/2
  Shift Arithmetic/1 -> Bitwise Operator1/2
  Mux/1 -> Out2/1
  Demux/3 -> Bitwise Operator2/1
  Shift Arithmetic1/1 -> Bitwise Operator2/2
  Shift Arithmetic2/1 -> Bitwise Operator3/2
  Demux/2 -> Shift Arithmetic/1
  Demux/4 -> Shift Arithmetic1/1
  Demux/6 -> Shift Arithmetic2/1
  Demux/1 -> Bitwise Operator1/1
  Demux/5 -> Bitwise Operator3/1
  Bitwise Operator/1 -> Demux/1
  Data Type Conversion/1 -> Bitwise Operator/1
  I2C Receive1/2 -> Terminator1/1
  I2C Receive1/1 -> Data Type Conversion/1

== system Deployed_On_CPU2/Subsystem3/Data acquisition/Reset3 ==
  function : TriggerPort  TriggerType=function-call  VariantControl=Variant
  Data Read Adress : Constant  Priority=10  Value=hex2dec('28')  OutDataTypeStr=uint8  SampleTime=-1
  I2C Transmit : c280xlib/I2C Transmit  Priority=20  selectModule=I2C_A  addrFormat=7-Bit addressing  saSource=Specify via dialog  SAR=hex2dec('69')  bitCount=8  STP=off  RM=off  STR=on
      settings: SourceProductBaseCode=TIC2000
  Terminator : Terminator
  wires:
  I2C Transmit/1 -> Terminator/1
  Data Read Adress/1 -> I2C Transmit/1

== system Deployed_On_CPU2/Subsystem3/Data acquisition/Reset4 ==
  function : TriggerPort  TriggerType=function-call  VariantControl=Variant
  Data Read Adress : Constant  Priority=10  Value=hex2dec('29')  OutDataTypeStr=uint8  SampleTime=-1
  I2C Transmit : c280xlib/I2C Transmit  Priority=20  selectModule=I2C_A  addrFormat=7-Bit addressing  saSource=Specify via dialog  SAR=hex2dec('69')  bitCount=8  STP=off  RM=off  STR=on
      settings: SourceProductBaseCode=TIC2000
  Terminator : Terminator
  wires:
  Data Read Adress/1 -> I2C Transmit/1
  I2C Transmit/1 -> Terminator/1

== system Deployed_On_CPU2/Subsystem3/Data acquisition/Reset5 ==
  function : TriggerPort  TriggerType=function-call  VariantControl=Variant
  Data Read Adress : Constant  Priority=10  Value=hex2dec('2A')  OutDataTypeStr=uint8  SampleTime=-1
  I2C Transmit : c280xlib/I2C Transmit  Priority=20  selectModule=I2C_A  addrFormat=7-Bit addressing  saSource=Specify via dialog  SAR=hex2dec('69')  bitCount=8  STP=off  RM=off  STR=on
      settings: SourceProductBaseCode=TIC2000
  Terminator : Terminator
  wires:
  I2C Transmit/1 -> Terminator/1
  Data Read Adress/1 -> I2C Transmit/1

== system Deployed_On_CPU2/Subsystem3/Data acquisition/Reset6 ==
  function : TriggerPort  TriggerType=function-call  VariantControl=Variant
  Data Read Adress : Constant  Priority=10  Value=hex2dec('2B')  OutDataTypeStr=uint8  SampleTime=-1
  I2C Transmit : c280xlib/I2C Transmit  Priority=20  selectModule=I2C_A  addrFormat=7-Bit addressing  saSource=Specify via dialog  SAR=hex2dec('69')  bitCount=8  STP=on  RM=off  STR=on
      settings: SourceProductBaseCode=TIC2000
  Terminator : Terminator
  wires:
  Data Read Adress/1 -> I2C Transmit/1
  I2C Transmit/1 -> Terminator/1

== system Deployed_On_CPU2/Subsystem3/Data acquisition/Reset7 ==
  function : TriggerPort  TriggerType=function-call  VariantControl=Variant
  Data Read Adress : Constant  Priority=10  Value=hex2dec('2C')  OutDataTypeStr=uint8  SampleTime=-1
  I2C Transmit : c280xlib/I2C Transmit  Priority=20  selectModule=I2C_A  addrFormat=7-Bit addressing  saSource=Specify via dialog  SAR=hex2dec('69')  bitCount=8  STP=off  RM=off  STR=on
      settings: SourceProductBaseCode=TIC2000
  Terminator : Terminator
  wires:
  I2C Transmit/1 -> Terminator/1
  Data Read Adress/1 -> I2C Transmit/1

== system Deployed_On_CPU2/Subsystem3/Data acquisition/Reset8 ==
  function : TriggerPort  TriggerType=function-call  VariantControl=Variant
  Data Read Adress : Constant  Priority=10  Value=hex2dec('2D')  OutDataTypeStr=uint8  SampleTime=-1
  I2C Transmit : c280xlib/I2C Transmit  Priority=20  selectModule=I2C_A  addrFormat=7-Bit addressing  saSource=Specify via dialog  SAR=hex2dec('69')  bitCount=8  STP=off  RM=off  STR=on
      settings: SourceProductBaseCode=TIC2000
  Terminator : Terminator
  wires:
  Data Read Adress/1 -> I2C Transmit/1
  I2C Transmit/1 -> Terminator/1
